simulink model "PAC Exp7"  (R2016a)
settings: Solver=VariableStepAuto  StartTime=0.0  StopTime=200  RelTol=1e-3
settings Model: Creator=PAPUN  LastModifiedBy=PAPUN

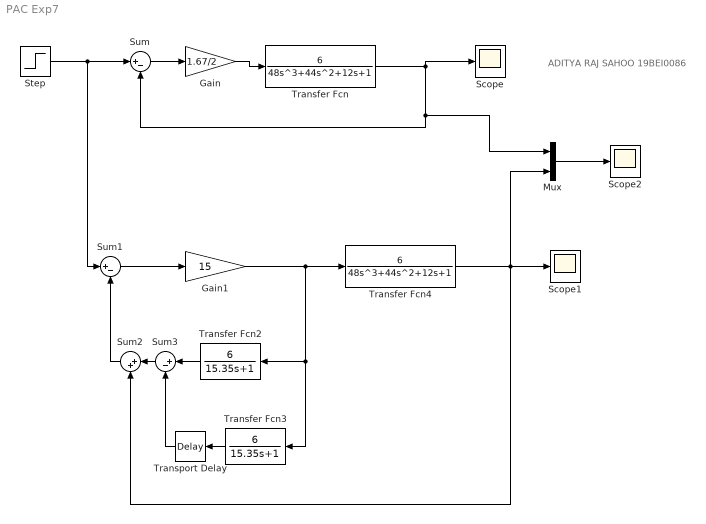
== system PAC Exp7 ==
  note: ADITYA RAJ SAHOO
      | 19BEI0086
  Gain : Gain  Gain=1.67/2
  Gain1 : Gain  Gain=15
  Mux : Mux  Inputs=2
  Scope : Scope
  Scope1 : Scope
  Scope2 : Scope
  Step : Step  SampleTime=0
  Sum : Sum  Inputs=|+-
  Sum1 : Sum  Inputs=|+-
  Sum2 : Sum  Inputs=|++
  Sum3 : Sum  Inputs=|+-
  Transfer Fcn : TransferFcn  Numerator=[6]  Denominator=[48 44 12 1]
  Transfer Fcn2 : TransferFcn  Numerator=[6]  Denominator=[15.35 1]
  Transfer Fcn3 : TransferFcn  Numerator=[6]  Denominator=[15.35 1]
  Transfer Fcn4 : TransferFcn  Numerator=[6]  Denominator=[48 44 12 1]
  Transport Delay : TransportDelay  DelayTime=2.71
  wires:
  Step/1 -> Sum1/1, Sum/1
  Sum/1 -> Gain/1
  Gain/1 -> Transfer Fcn/1
  Sum1/1 -> Gain1/1
  Transfer Fcn/1 -> Scope/1, Mux/1, Sum/2
  Mux/1 -> Scope2/1
  Transfer Fcn2/1 -> Sum3/1
  Sum3/1 -> Sum2/1
  Sum2/1 -> Sum1/2
  Transfer Fcn3/1 -> Transport Delay/1
  Transport Delay/1 -> Sum3/2
  Gain1/1 -> Transfer Fcn4/1, Transfer Fcn3/1, Transfer Fcn2/1
  Transfer Fcn4/1 -> Scope1/1, Sum2/2, Mux/2
